simulink model "gm_spectrum_analyser"  (R2020a)
settings: Solver=VariableStepAuto  StartTime=0.0  StopTime=100000/256e6  RelTol=1e-3
InitFcn:
  | fs = 256e6;
undefined symbols (not defined in the file or in its folder): designMultirateFIR
libraries: hdlsllib x81, simulink x50, dspmlti4 x6, dsphdlxfrm x5, hdlmdlgenlib x4, dspswit3 x4, dspsigops x2, dspsigattribs x2
(part 4 of 5)

== system gm_spectrum_analyser/Spectrum Analyser/Spectrum Analyser/Spectrum Analyser Core/Preprocessing Window/Direct Memory Access/DDR Read Controller ==
  length_in : Inport  OutDataTypeStr=uint32  PortDimensions=1  SampleTime=3.90625e-09
  address : Inport  Port=2  OutDataTypeStr=uint32  PortDimensions=1  SampleTime=3.90625e-09
  start : Inport  Port=3  OutDataTypeStr=boolean  PortDimensions=1  SampleTime=3.90625e-09
  rd_aready : Inport  Port=4  OutDataTypeStr=boolean  PortDimensions=1  SampleTime=3.90625e-09
  rd_dvalid : Inport  Port=5  OutDataTypeStr=boolean  PortDimensions=1  SampleTime=3.90625e-09
  slib_spectrum_analyser_c5_DDR_Read_Controller : MATLAB Function  TreatAsAtomicUnit=on
  valid_out : Outport  VectorParamsAs1DForOutWhenUnconnected=off
  count_out : Outport  Port=2  VectorParamsAs1DForOutWhenUnconnected=off
  ready_out : Outport  Port=3  VectorParamsAs1DForOutWhenUnconnected=off
  rd_addr : Outport  Port=4  VectorParamsAs1DForOutWhenUnconnected=off
  rd_len : Outport  Port=5  VectorParamsAs1DForOutWhenUnconnected=off
  rd_avalid : Outport  Port=6  VectorParamsAs1DForOutWhenUnconnected=off
  wires:
  slib_spectrum_analyser_c5_DDR_Read_Controller/1(valid_out) -> valid_out/1
  slib_spectrum_analyser_c5_DDR_Read_Controller/2(count_out) -> count_out/1
  slib_spectrum_analyser_c5_DDR_Read_Controller/3(ready_out) -> ready_out/1
  slib_spectrum_analyser_c5_DDR_Read_Controller/4(rd_addr) -> rd_addr/1
  slib_spectrum_analyser_c5_DDR_Read_Controller/5(rd_len) -> rd_len/1
  slib_spectrum_analyser_c5_DDR_Read_Controller/6(rd_avalid) -> rd_avalid/1
  length_in/1 -> slib_spectrum_analyser_c5_DDR_Read_Controller/1(length_in)
  address/1 -> slib_spectrum_analyser_c5_DDR_Read_Controller/2(address)
  start/1 -> slib_spectrum_analyser_c5_DDR_Read_Controller/3(start)
  rd_aready/1 -> slib_spectrum_analyser_c5_DDR_Read_Controller/4(rd_aready)
  rd_dvalid/1 -> slib_spectrum_analyser_c5_DDR_Read_Controller/5(rd_dvalid)

== system gm_spectrum_analyser/Spectrum Analyser/Spectrum Analyser/Spectrum Analyser Core/Preprocessing Window/Direct Memory Access/EdgeDetection ==
  In1 : Inport  OutDataTypeStr=fixdt(0, 1, 0)  PortDimensions=1  SampleTime=3.90625e-09
  Delay : Delay  DelayLength=double(1)  InitialCondition=0  SampleTime=3.90625e-09
  Logical Operator : Logic  AllPortsSameDT=off  OutDataTypeStr=boolean  SampleTime=3.90625e-09
  Logical Operator1 : Logic  Operator=NOT  Inputs=1  AllPortsSameDT=off  OutDataTypeStr=boolean  SampleTime=3.90625e-09
  Out1 : Outport  VectorParamsAs1DForOutWhenUnconnected=off
  wires:
  Delay/1 -> Logical Operator1/1
  Logical Operator/1 -> Out1/1
  Logical Operator1/1 -> Logical Operator/1
  In1/1 -> Logical Operator/2, Delay/1

== system gm_spectrum_analyser/Spectrum Analyser/Spectrum Analyser/Spectrum Analyser Core/SSR Subset Converter/SSR Deserializer Imag/SSR to Vector ==
  SSR : Inport  OutDataTypeStr=fixdt(0, 128, 0)  PortDimensions=1  SampleTime=3.90625e-09
  Bit Slice0 : hdlsllib/Logic and Bit Operations/Bit Slice  lidx=double(15)  ridx=double(0)
      settings: SourceProductBaseCode=SL
  Bit Slice1 : hdlsllib/Logic and Bit Operations/Bit Slice  lidx=double(31)  ridx=double(16)
      settings: SourceProductBaseCode=SL
  Bit Slice2 : hdlsllib/Logic and Bit Operations/Bit Slice  lidx=double(47)  ridx=double(32)
      settings: SourceProductBaseCode=SL
  Bit Slice3 : hdlsllib/Logic and Bit Operations/Bit Slice  lidx=double(63)  ridx=double(48)
      settings: SourceProductBaseCode=SL
  Bit Slice4 : hdlsllib/Logic and Bit Operations/Bit Slice  lidx=double(79)  ridx=double(64)
      settings: SourceProductBaseCode=SL
  Bit Slice5 : hdlsllib/Logic and Bit Operations/Bit Slice  lidx=double(95)  ridx=double(80)
      settings: SourceProductBaseCode=SL
  Bit Slice6 : hdlsllib/Logic and Bit Operations/Bit Slice  lidx=double(111)  ridx=double(96)
      settings: SourceProductBaseCode=SL
  Bit Slice7 : hdlsllib/Logic and Bit Operations/Bit Slice  lidx=double(127)  ridx=double(112)
      settings: SourceProductBaseCode=SL
  concatenate : Concatenate  NumInputs=8
  Vector : Outport
  wires:
  Bit Slice0/1 -> concatenate/1
  Bit Slice1/1 -> concatenate/2
  Bit Slice2/1 -> concatenate/3
  Bit Slice3/1 -> concatenate/4
  Bit Slice4/1 -> concatenate/5
  Bit Slice5/1 -> concatenate/6
  Bit Slice6/1 -> concatenate/7
  Bit Slice7/1 -> concatenate/8
  concatenate/1 -> Vector/1
  SSR/1 -> Bit Slice7/1, Bit Slice6/1, Bit Slice5/1, Bit Slice4/1, Bit Slice3/1, Bit Slice2/1, Bit Slice1/1, Bit Slice0/1

== system gm_spectrum_analyser/Spectrum Analyser/Spectrum Analyser/Spectrum Analyser Core/SSR Subset Converter/SSR Deserializer Imag/Subsystem ==
  Set : Inport  OutDataTypeStr=boolean  PortDimensions=1  SampleTime=3.90625e-09
  Reset : Inport  Port=2  OutDataTypeStr=boolean  PortDimensions=1  SampleTime=3.90625e-09
  Constant : Constant  OutDataTypeStr=boolean  SampleTime=3.90625e-09
  Initial_Val : Constant  Value=double(0)  OutDataTypeStr=boolean  SampleTime=3.90625e-09
  Multiport Switch : MultiPortSwitch  DataPortOrder=Zero-based contiguous  Inputs=2  DiagnosticForDefault=None  zeroidx=on  SampleTime=3.90625e-09
  Unit Delay Resettable Synchronous_lowered : Delay  DelayLength=double(1)  InitialCondition=0  SampleTime=3.90625e-09
  reset_in : Switch  Criteria=u2 ~= 0  Threshold=double(0)  OutDataTypeStr=boolean  SampleTime=3.90625e-09
  Latch : Outport
  wires:
  Constant/1 -> Multiport Switch/3
  Multiport Switch/1 -> Latch/1, reset_in/3
  Initial_Val/1 -> reset_in/1
  Set/1 -> Multiport Switch/1
  Reset/1 -> reset_in/2
  reset_in/1 -> Unit Delay Resettable Synchronous_lowered/1
  Unit Delay Resettable Synchronous_lowered/1 -> Multiport Switch/2

== system gm_spectrum_analyser/Spectrum Analyser/Spectrum Analyser/Spectrum Analyser Core/SSR Subset Converter/SSR Deserializer Imag/Subsystem1 ==
  Set : Inport  OutDataTypeStr=boolean  PortDimensions=1  SampleTime=3.90625e-09
  Reset : Inport  Port=2  OutDataTypeStr=boolean  PortDimensions=1  SampleTime=3.90625e-09
  Constant : Constant  OutDataTypeStr=boolean  SampleTime=3.90625e-09
  Initial_Val : Constant  Value=double(0)  OutDataTypeStr=boolean  SampleTime=3.90625e-09
  Multiport Switch : MultiPortSwitch  DataPortOrder=Zero-based contiguous  Inputs=2  DiagnosticForDefault=None  zeroidx=on  SampleTime=3.90625e-09
  Unit Delay Resettable Synchronous_lowered : Delay  DelayLength=double(1)  InitialCondition=0  SampleTime=3.90625e-09
  reset_in : Switch  Criteria=u2 ~= 0  Threshold=double(0)  OutDataTypeStr=boolean  SampleTime=3.90625e-09
  Latch : Outport
  wires:
  Constant/1 -> Multiport Switch/3
  Multiport Switch/1 -> Latch/1, reset_in/3
  Initial_Val/1 -> reset_in/1
  Set/1 -> Multiport Switch/1
  Reset/1 -> reset_in/2
  reset_in/1 -> Unit Delay Resettable Synchronous_lowered/1
  Unit Delay Resettable Synchronous_lowered/1 -> Multiport Switch/2

== system gm_spectrum_analyser/Spectrum Analyser/Spectrum Analyser/Spectrum Analyser Core/SSR Subset Converter/SSR Deserializer Real/SSR to Vector ==
  SSR : Inport  OutDataTypeStr=fixdt(0, 128, 0)  PortDimensions=1  SampleTime=3.90625e-09
  Bit Slice0 : hdlsllib/Logic and Bit Operations/Bit Slice  lidx=double(15)  ridx=double(0)
      settings: SourceProductBaseCode=SL
  Bit Slice1 : hdlsllib/Logic and Bit Operations/Bit Slice  lidx=double(31)  ridx=double(16)
      settings: SourceProductBaseCode=SL
  Bit Slice2 : hdlsllib/Logic and Bit Operations/Bit Slice  lidx=double(47)  ridx=double(32)
      settings: SourceProductBaseCode=SL
  Bit Slice3 : hdlsllib/Logic and Bit Operations/Bit Slice  lidx=double(63)  ridx=double(48)
      settings: SourceProductBaseCode=SL
  Bit Slice4 : hdlsllib/Logic and Bit Operations/Bit Slice  lidx=double(79)  ridx=double(64)
      settings: SourceProductBaseCode=SL
  Bit Slice5 : hdlsllib/Logic and Bit Operations/Bit Slice  lidx=double(95)  ridx=double(80)
      settings: SourceProductBaseCode=SL
  Bit Slice6 : hdlsllib/Logic and Bit Operations/Bit Slice  lidx=double(111)  ridx=double(96)
      settings: SourceProductBaseCode=SL
  Bit Slice7 : hdlsllib/Logic and Bit Operations/Bit Slice  lidx=double(127)  ridx=double(112)
      settings: SourceProductBaseCode=SL
  concatenate : Concatenate  NumInputs=8
  Vector : Outport
  wires:
  Bit Slice0/1 -> concatenate/1
  Bit Slice1/1 -> concatenate/2
  Bit Slice2/1 -> concatenate/3
  Bit Slice3/1 -> concatenate/4
  Bit Slice4/1 -> concatenate/5
  Bit Slice5/1 -> concatenate/6
  Bit Slice6/1 -> concatenate/7
  Bit Slice7/1 -> concatenate/8
  concatenate/1 -> Vector/1
  SSR/1 -> Bit Slice7/1, Bit Slice6/1, Bit Slice5/1, Bit Slice4/1, Bit Slice3/1, Bit Slice2/1, Bit Slice1/1, Bit Slice0/1

== system gm_spectrum_analyser/Spectrum Analyser/Spectrum Analyser/Spectrum Analyser Core/SSR Subset Converter/SSR Deserializer Real/Subsystem ==
  Set : Inport  OutDataTypeStr=boolean  PortDimensions=1  SampleTime=3.90625e-09
  Reset : Inport  Port=2  OutDataTypeStr=boolean  PortDimensions=1  SampleTime=3.90625e-09
  Constant : Constant  OutDataTypeStr=boolean  SampleTime=3.90625e-09
  Initial_Val : Constant  Value=double(0)  OutDataTypeStr=boolean  SampleTime=3.90625e-09
  Multiport Switch : MultiPortSwitch  DataPortOrder=Zero-based contiguous  Inputs=2  DiagnosticForDefault=None  zeroidx=on  SampleTime=3.90625e-09
  Unit Delay Resettable Synchronous_lowered : Delay  DelayLength=double(1)  InitialCondition=0  SampleTime=3.90625e-09
  reset_in : Switch  Criteria=u2 ~= 0  Threshold=double(0)  OutDataTypeStr=boolean  SampleTime=3.90625e-09
  Latch : Outport
  wires:
  Constant/1 -> Multiport Switch/3
  Multiport Switch/1 -> Latch/1, reset_in/3
  Initial_Val/1 -> reset_in/1
  Set/1 -> Multiport Switch/1
  Reset/1 -> reset_in/2
  reset_in/1 -> Unit Delay Resettable Synchronous_lowered/1
  Unit Delay Resettable Synchronous_lowered/1 -> Multiport Switch/2

== system gm_spectrum_analyser/Spectrum Analyser/Spectrum Analyser/Spectrum Analyser Core/SSR Subset Converter/SSR Deserializer Real/Subsystem1 ==
  Set : Inport  OutDataTypeStr=boolean  PortDimensions=1  SampleTime=3.90625e-09
  Reset : Inport  Port=2  OutDataTypeStr=boolean  PortDimensions=1  SampleTime=3.90625e-09
  Constant : Constant  OutDataTypeStr=boolean  SampleTime=3.90625e-09
  Initial_Val : Constant  Value=double(0)  OutDataTypeStr=boolean  SampleTime=3.90625e-09
  Multiport Switch : MultiPortSwitch  DataPortOrder=Zero-based contiguous  Inputs=2  DiagnosticForDefault=None  zeroidx=on  SampleTime=3.90625e-09
  Unit Delay Resettable Synchronous_lowered : Delay  DelayLength=double(1)  InitialCondition=0  SampleTime=3.90625e-09
  reset_in : Switch  Criteria=u2 ~= 0  Threshold=double(0)  OutDataTypeStr=boolean  SampleTime=3.90625e-09
  Latch : Outport
  wires:
  Constant/1 -> Multiport Switch/3
  Multiport Switch/1 -> Latch/1, reset_in/3
  Initial_Val/1 -> reset_in/1
  Set/1 -> Multiport Switch/1
  Reset/1 -> reset_in/2
  reset_in/1 -> Unit Delay Resettable Synchronous_lowered/1
  Unit Delay Resettable Synchronous_lowered/1 -> Multiport Switch/2

== system gm_spectrum_analyser/Spectrum Analyser/Spectrum Analyser/Spectrum Analyser Core/SSR Subset Converter/SSR Packet Generator Imag/Frame Dropper ==
  Valid In : Inport  OutDataTypeStr=boolean  PortDimensions=1  SampleTime=3.90625e-09
  Data In : Inport  Port=2  OutDataTypeStr=fixdt(0, 128, 0)  PortDimensions=1  SampleTime=3.90625e-09
  SoF In : Inport  Port=3  OutDataTypeStr=boolean  PortDimensions=1  SampleTime=3.90625e-09
  EoF In : Inport  Port=4  OutDataTypeStr=boolean  PortDimensions=1  SampleTime=3.90625e-09
  Frame Drop : Inport  Port=5  OutDataTypeStr=fixdt(0, 4, 0)  PortDimensions=1  SampleTime=3.90625e-09
  AND : Logic  AllPortsSameDT=off  OutDataTypeStr=boolean  SampleTime=3.90625e-09
  AND1 : Logic  AllPortsSameDT=off  OutDataTypeStr=boolean  SampleTime=3.90625e-09
  AND2 : Logic  AllPortsSameDT=off  OutDataTypeStr=boolean  SampleTime=3.90625e-09
  Compare To Zero : simulink/Logic and Bit Operations/Compare To Constant  relop===  const=double(0)  OutDataTypeStr=boolean
  Constant : Constant  Value=0  OutDataTypeStr=fixdt(0, 4, 0)  SampleTime=3.90625e-09
  Constant1 : Constant  OutDataTypeStr=fixdt(0, 4, 0)  SampleTime=3.90625e-09
  HDL Counter : hdlsllib/Sources/HDL Counter  CountType=Count limited  CountInit=double(0)  CountStep=double(1)  CountMax=double(7)  CountFromType=Initial value  CountFrom=double(0)  CountResetPort=on  CountLoadPort=off  CountEnbPort=on  CountDirPort=off  CountDataType=Unsigned  CountWordLen=4  CountFracLen=0  CountSampTime=3.90625e-09
  Multiport Switch : MultiPortSwitch  DataPortOrder=Zero-based contiguous  Inputs=2  DiagnosticForDefault=None  zeroidx=on  OutDataTypeStr=fixdt(0, 4, 0)  SampleTime=3.90625e-09
  Relational Operator : RelationalOperator  Operator=<=  OutDataTypeStr=boolean  SampleTime=3.90625e-09  RndMeth=Nearest
  shift arithmetic : ArithShift  BitShiftNumberSource=Input port  BitShiftDirection=Left
      settings: InputPortMap=u0,p1
  Valid Out : Outport
  Data Out : Outport  Port=2
  SoF Out : Outport  Port=3
  EoF Out : Outport  Port=4
  wires:
  AND/1 -> Valid Out/1
  AND1/1 -> EoF Out/1
  AND2/1 -> SoF Out/1
  Compare To Zero/1 -> AND2/1, AND1/1, AND/2
  Constant/1 -> Multiport Switch/3
  Constant1/1 -> shift arithmetic/1
  HDL Counter/1 -> Multiport Switch/2, Relational Operator/2
  Multiport Switch/1 -> Compare To Zero/1
  Relational Operator/1 -> Multiport Switch/1, HDL Counter/1
  shift arithmetic/1 -> Relational Operator/1
  Valid In/1 -> AND/1
  Data In/1 -> Data Out/1
  SoF In/1 -> AND2/2
  EoF In/1 -> AND1/2, HDL Counter/2
  Frame Drop/1 -> shift arithmetic/2

== system gm_spectrum_analyser/Spectrum Analyser/Spectrum Analyser/Spectrum Analyser Core/SSR Subset Converter/SSR Packet Generator Imag/TLAST Generator ==
  Valid In : Inport  OutDataTypeStr=boolean  PortDimensions=1  SampleTime=3.90625e-09
  Data In : Inport  Port=2  OutDataTypeStr=fixdt(0, 128, 0)  PortDimensions=1  SampleTime=3.90625e-09
  Packet Size : Inport  Port=3  OutDataTypeStr=uint32  PortDimensions=1  SampleTime=3.90625e-09
  AND : Logic  Inputs=3  AllPortsSameDT=off  OutDataTypeStr=boolean  SampleTime=3.90625e-09
  AND1 : Logic  Inputs=3  AllPortsSameDT=off  OutDataTypeStr=boolean  SampleTime=3.90625e-09
  AND2 : Logic  AllPortsSameDT=off  OutDataTypeStr=boolean  SampleTime=3.90625e-09
  AND3 : Logic  AllPortsSameDT=off  OutDataTypeStr=boolean  SampleTime=3.90625e-09
  Compare To Constant : simulink/Logic and Bit Operations/Compare To Constant  relop===  const="fi(0,0,32,0,\"hex\",\"00000001\")"  OutDataTypeStr=boolean
  Compare To Zero : simulink/Logic and Bit Operations/Compare To Constant  relop=~=  const=double(0)  OutDataTypeStr=boolean
  Delay_Switch : Switch  Criteria=u2 ~= 0  Threshold=double(0)  OutDataTypeStr=uint32  SampleTime=3.90625e-09
  HDL Counter : hdlsllib/Sources/HDL Counter  CountType=Free running  CountInit=double(1)  CountStep=double(1)  CountMax=25  CountFromType=Initial value  CountFrom=double(1)  CountResetPort=on  CountLoadPort=off  CountEnbPort=on  CountDirPort=off  CountDataType=Unsigned  CountWordLen=32  CountFracLen=0  CountSampTime=3.90625e-09
  Relational Operator : RelationalOperator  Operator=<=  OutDataTypeStr=boolean  SampleTime=3.90625e-09  RndMeth=Nearest
  Unit Delay Enabled Synchronous_lowered : Delay  DelayLength=double(1)  InitialCondition=0  SampleTime=3.90625e-09
  Valid Out : Outport
  Data Out : Outport  Port=2
  SoF Out : Outport  Port=3
  EoF Out : Outport  Port=4
  wires:
  AND/1 -> SoF Out/1
  AND1/1 -> EoF Out/1, HDL Counter/1
  AND2/1 -> Valid Out/1
  Compare To Constant/1 -> AND/1
  Compare To Zero/1 -> AND2/1, AND/3, AND1/3
  HDL Counter/1 -> Compare To Constant/1, Relational Operator/2
  Valid In/1 -> AND2/2, AND/2, AND3/1, AND1/2, HDL Counter/2
  Data In/1 -> Data Out/1
  Packet Size/1 -> Delay_Switch/1
  Relational Operator/1 -> AND3/2, AND1/1
  AND3/1 -> Delay_Switch/2
  Delay_Switch/1 -> Unit Delay Enabled Synchronous_lowered/1
  Unit Delay Enabled Synchronous_lowered/1 -> Relational Operator/1, Compare To Zero/1, Delay_Switch/3

== system gm_spectrum_analyser/Spectrum Analyser/Spectrum Analyser/Spectrum Analyser Core/SSR Subset Converter/SSR Packet Generator Real/Frame Dropper ==
  Valid In : Inport  OutDataTypeStr=boolean  PortDimensions=1  SampleTime=3.90625e-09
  Data In : Inport  Port=2  OutDataTypeStr=fixdt(0, 128, 0)  PortDimensions=1  SampleTime=3.90625e-09
  SoF In : Inport  Port=3  OutDataTypeStr=boolean  PortDimensions=1  SampleTime=3.90625e-09
  EoF In : Inport  Port=4  OutDataTypeStr=boolean  PortDimensions=1  SampleTime=3.90625e-09
  Frame Drop : Inport  Port=5  OutDataTypeStr=fixdt(0, 4, 0)  PortDimensions=1  SampleTime=3.90625e-09
  AND : Logic  AllPortsSameDT=off  OutDataTypeStr=boolean  SampleTime=3.90625e-09
  AND1 : Logic  AllPortsSameDT=off  OutDataTypeStr=boolean  SampleTime=3.90625e-09
  AND2 : Logic  AllPortsSameDT=off  OutDataTypeStr=boolean  SampleTime=3.90625e-09
  Compare To Zero : simulink/Logic and Bit Operations/Compare To Constant  relop===  const=double(0)  OutDataTypeStr=boolean
  Constant : Constant  Value=0  OutDataTypeStr=fixdt(0, 4, 0)  SampleTime=3.90625e-09
  Constant1 : Constant  OutDataTypeStr=fixdt(0, 4, 0)  SampleTime=3.90625e-09
  HDL Counter : hdlsllib/Sources/HDL Counter  CountType=Count limited  CountInit=double(0)  CountStep=double(1)  CountMax=double(7)  CountFromType=Initial value  CountFrom=double(0)  CountResetPort=on  CountLoadPort=off  CountEnbPort=on  CountDirPort=off  CountDataType=Unsigned  CountWordLen=4  CountFracLen=0  CountSampTime=3.90625e-09
  Multiport Switch : MultiPortSwitch  DataPortOrder=Zero-based contiguous  Inputs=2  DiagnosticForDefault=None  zeroidx=on  OutDataTypeStr=fixdt(0, 4, 0)  SampleTime=3.90625e-09
  Relational Operator : RelationalOperator  Operator=<=  OutDataTypeStr=boolean  SampleTime=3.90625e-09  RndMeth=Nearest
  shift arithmetic : ArithShift  BitShiftNumberSource=Input port  BitShiftDirection=Left
      settings: InputPortMap=u0,p1
  Valid Out : Outport
  Data Out : Outport  Port=2
  SoF Out : Outport  Port=3
  EoF Out : Outport  Port=4
  wires:
  AND/1 -> Valid Out/1
  AND1/1 -> EoF Out/1
  AND2/1 -> SoF Out/1
  Compare To Zero/1 -> AND2/1, AND1/1, AND/2
  Constant/1 -> Multiport Switch/3
  Constant1/1 -> shift arithmetic/1
  HDL Counter/1 -> Multiport Switch/2, Relational Operator/2
  Multiport Switch/1 -> Compare To Zero/1
  Relational Operator/1 -> Multiport Switch/1, HDL Counter/1
  shift arithmetic/1 -> Relational Operator/1
  Valid In/1 -> AND/1
  Data In/1 -> Data Out/1
  SoF In/1 -> AND2/2
  EoF In/1 -> AND1/2, HDL Counter/2
  Frame Drop/1 -> shift arithmetic/2

== system gm_spectrum_analyser/Spectrum Analyser/Spectrum Analyser/Spectrum Analyser Core/SSR Subset Converter/SSR Packet Generator Real/TLAST Generator ==
  Valid In : Inport  OutDataTypeStr=boolean  PortDimensions=1  SampleTime=3.90625e-09
  Data In : Inport  Port=2  OutDataTypeStr=fixdt(0, 128, 0)  PortDimensions=1  SampleTime=3.90625e-09
  Packet Size : Inport  Port=3  OutDataTypeStr=uint32  PortDimensions=1  SampleTime=3.90625e-09
  AND : Logic  Inputs=3  AllPortsSameDT=off  OutDataTypeStr=boolean  SampleTime=3.90625e-09
  AND1 : Logic  Inputs=3  AllPortsSameDT=off  OutDataTypeStr=boolean  SampleTime=3.90625e-09
  AND2 : Logic  AllPortsSameDT=off  OutDataTypeStr=boolean  SampleTime=3.90625e-09
  AND3 : Logic  AllPortsSameDT=off  OutDataTypeStr=boolean  SampleTime=3.90625e-09
  Compare To Constant : simulink/Logic and Bit Operations/Compare To Constant  relop===  const="fi(0,0,32,0,\"hex\",\"00000001\")"  OutDataTypeStr=boolean
  Compare To Zero : simulink/Logic and Bit Operations/Compare To Constant  relop=~=  const=double(0)  OutDataTypeStr=boolean
  Delay_Switch : Switch  Criteria=u2 ~= 0  Threshold=double(0)  OutDataTypeStr=uint32  SampleTime=3.90625e-09
  HDL Counter : hdlsllib/Sources/HDL Counter  CountType=Free running  CountInit=double(1)  CountStep=double(1)  CountMax=25  CountFromType=Initial value  CountFrom=double(1)  CountResetPort=on  CountLoadPort=off  CountEnbPort=on  CountDirPort=off  CountDataType=Unsigned  CountWordLen=32  CountFracLen=0  CountSampTime=3.90625e-09
  Relational Operator : RelationalOperator  Operator=<=  OutDataTypeStr=boolean  SampleTime=3.90625e-09  RndMeth=Nearest
  Unit Delay Enabled Synchronous_lowered : Delay  DelayLength=double(1)  InitialCondition=0  SampleTime=3.90625e-09
  Valid Out : Outport
  Data Out : Outport  Port=2
  SoF Out : Outport  Port=3
  EoF Out : Outport  Port=4
  wires:
  AND/1 -> SoF Out/1
  AND1/1 -> EoF Out/1, HDL Counter/1
  AND2/1 -> Valid Out/1
  Compare To Constant/1 -> AND/1
  Compare To Zero/1 -> AND2/1, AND/3, AND1/3
  HDL Counter/1 -> Compare To Constant/1, Relational Operator/2
  Valid In/1 -> AND2/2, AND/2, AND3/1, AND1/2, HDL Counter/2
  Data In/1 -> Data Out/1
  Packet Size/1 -> Delay_Switch/1
  Relational Operator/1 -> AND3/2, AND1/1
  AND3/1 -> Delay_Switch/2
  Delay_Switch/1 -> Unit Delay Enabled Synchronous_lowered/1
  Unit Delay Enabled Synchronous_lowered/1 -> Relational Operator/1, Compare To Zero/1, Delay_Switch/3

== system gm_spectrum_analyser/Spectrum Analyser/Spectrum Analyser/Spectrum Analyser Core/SSR Subset Converter/SSR Serializer Imag/SSR to Vector ==
  SSR : Inport  OutDataTypeStr=fixdt(0, 128, 0)  PortDimensions=1  SampleTime=3.90625e-09
  Bit Slice0 : hdlsllib/Logic and Bit Operations/Bit Slice  lidx=double(15)  ridx=double(0)
      settings: SourceProductBaseCode=SL
  Bit Slice1 : hdlsllib/Logic and Bit Operations/Bit Slice  lidx=double(31)  ridx=double(16)
      settings: SourceProductBaseCode=SL
  Bit Slice2 : hdlsllib/Logic and Bit Operations/Bit Slice  lidx=double(47)  ridx=double(32)
      settings: SourceProductBaseCode=SL
  Bit Slice3 : hdlsllib/Logic and Bit Operations/Bit Slice  lidx=double(63)  ridx=double(48)
      settings: SourceProductBaseCode=SL
  Bit Slice4 : hdlsllib/Logic and Bit Operations/Bit Slice  lidx=double(79)  ridx=double(64)
      settings: SourceProductBaseCode=SL
  Bit Slice5 : hdlsllib/Logic and Bit Operations/Bit Slice  lidx=double(95)  ridx=double(80)
      settings: SourceProductBaseCode=SL
  Bit Slice6 : hdlsllib/Logic and Bit Operations/Bit Slice  lidx=double(111)  ridx=double(96)
      settings: SourceProductBaseCode=SL
  Bit Slice7 : hdlsllib/Logic and Bit Operations/Bit Slice  lidx=double(127)  ridx=double(112)
      settings: SourceProductBaseCode=SL
  concatenate : Concatenate  NumInputs=8
  Vector : Outport
  wires:
  Bit Slice0/1 -> concatenate/1
  Bit Slice1/1 -> concatenate/2
  Bit Slice2/1 -> concatenate/3
  Bit Slice3/1 -> concatenate/4
  Bit Slice4/1 -> concatenate/5
  Bit Slice5/1 -> concatenate/6
  Bit Slice6/1 -> concatenate/7
  Bit Slice7/1 -> concatenate/8
  concatenate/1 -> Vector/1
  SSR/1 -> Bit Slice7/1, Bit Slice6/1, Bit Slice5/1, Bit Slice4/1, Bit Slice3/1, Bit Slice2/1, Bit Slice1/1, Bit Slice0/1

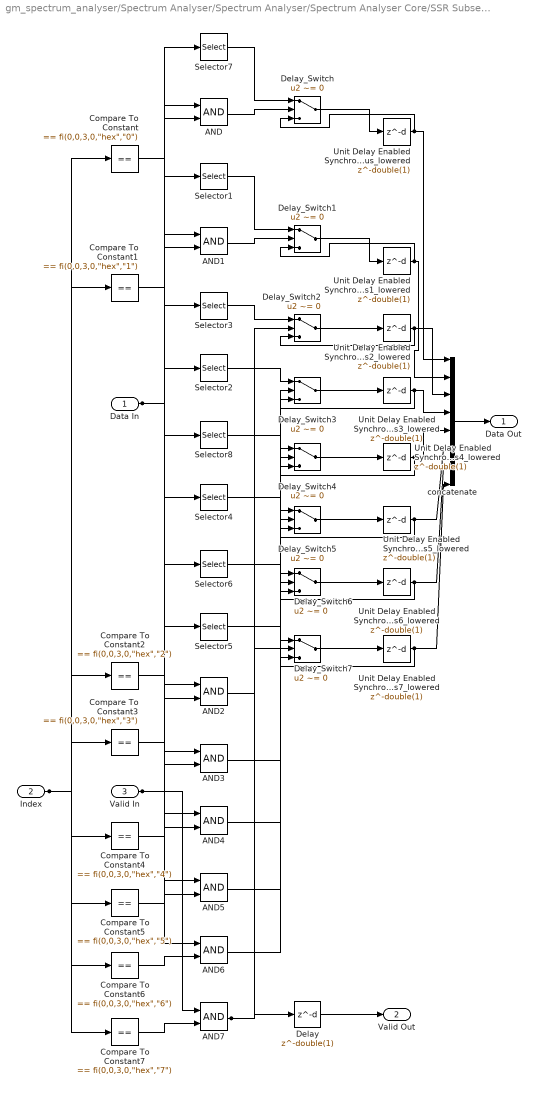
== system gm_spectrum_analyser/Spectrum Analyser/Spectrum Analyser/Spectrum Analyser Core/SSR Subset Converter/SSR Serializer Imag/SSR1 to SSR8 ==
  Data In : Inport  OutDataTypeStr=uint16  PortDimensions=[8]  SampleTime=3.90625e-09
  Index : Inport  Port=2  OutDataTypeStr=fixdt(0, 3, 0)  PortDimensions=1  SampleTime=3.90625e-09
  Valid In : Inport  Port=3  OutDataTypeStr=boolean  PortDimensions=1  SampleTime=3.90625e-09
  AND{,1..7} (8 alike) : Logic  AllPortsSameDT=off  OutDataTypeStr=boolean  SampleTime=3.90625e-09
  Compare To Constant : simulink/Logic and Bit Operations/Compare To Constant  relop===  const="fi(0,0,3,0,\"hex\",\"0\")"  OutDataTypeStr=boolean
  Compare To Constant1 : simulink/Logic and Bit Operations/Compare To Constant  relop===  const="fi(0,0,3,0,\"hex\",\"1\")"  OutDataTypeStr=boolean
  Compare To Constant2 : simulink/Logic and Bit Operations/Compare To Constant  relop===  const="fi(0,0,3,0,\"hex\",\"2\")"  OutDataTypeStr=boolean
  Compare To Constant3 : simulink/Logic and Bit Operations/Compare To Constant  relop===  const="fi(0,0,3,0,\"hex\",\"3\")"  OutDataTypeStr=boolean
  Compare To Constant4 : simulink/Logic and Bit Operations/Compare To Constant  relop===  const="fi(0,0,3,0,\"hex\",\"4\")"  OutDataTypeStr=boolean
  Compare To Constant5 : simulink/Logic and Bit Operations/Compare To Constant  relop===  const="fi(0,0,3,0,\"hex\",\"5\")"  OutDataTypeStr=boolean
  Compare To Constant6 : simulink/Logic and Bit Operations/Compare To Constant  relop===  const="fi(0,0,3,0,\"hex\",\"6\")"  OutDataTypeStr=boolean
  Compare To Constant7 : simulink/Logic and Bit Operations/Compare To Constant  relop===  const="fi(0,0,3,0,\"hex\",\"7\")"  OutDataTypeStr=boolean
  Delay : Delay  DelayLength=double(1)  InitialCondition=0  SampleTime=3.90625e-09
  Delay_Switch{,1..7} (8 alike) : Switch  Criteria=u2 ~= 0  Threshold=double(0)  OutDataTypeStr=uint16  SampleTime=3.90625e-09
  Selector{1..8} (8 alike) : Selector  IndexMode=Zero-based  SampleTime=3.90625e-09  IndexOptions=Index vector (dialog)  Indices=double(0)  OutputSizes=double(1)
  Unit Delay Enabled Synchronous1_lowered : Delay  DelayLength=double(1)  InitialCondition=0  SampleTime=3.90625e-09
  Unit Delay Enabled Synchronous2_lowered : Delay  DelayLength=double(1)  InitialCondition=0  SampleTime=3.90625e-09
  Unit Delay Enabled Synchronous3_lowered : Delay  DelayLength=double(1)  InitialCondition=0  SampleTime=3.90625e-09
  Unit Delay Enabled Synchronous4_lowered : Delay  DelayLength=double(1)  InitialCondition=0  SampleTime=3.90625e-09
  Unit Delay Enabled Synchronous5_lowered : Delay  DelayLength=double(1)  InitialCondition=0  SampleTime=3.90625e-09
  Unit Delay Enabled Synchronous6_lowered : Delay  DelayLength=double(1)  InitialCondition=0  SampleTime=3.90625e-09
  Unit Delay Enabled Synchronous7_lowered : Delay  DelayLength=double(1)  InitialCondition=0  SampleTime=3.90625e-09
  Unit Delay Enabled Synchronous_lowered : Delay  DelayLength=double(1)  InitialCondition=0  SampleTime=3.90625e-09
  concatenate : Concatenate  NumInputs=8
  Data Out : Outport
  Valid Out : Outport  Port=2
  wires:
  AND/1 -> Delay_Switch/2
  AND1/1 -> Delay_Switch1/2
  AND2/1 -> Delay_Switch2/2
  AND3/1 -> Delay_Switch3/2
  AND4/1 -> Delay_Switch4/2
  AND5/1 -> Delay_Switch5/2
  AND6/1 -> Delay_Switch6/2
  AND7/1 -> Delay/1, Delay_Switch7/2
  Compare To Constant/1 -> AND/2
  Compare To Constant1/1 -> AND1/2
  Compare To Constant2/1 -> AND2/2
  Compare To Constant3/1 -> AND3/2
  Compare To Constant4/1 -> AND4/2
  Compare To Constant5/1 -> AND5/2
  Compare To Constant6/1 -> AND6/2
  Compare To Constant7/1 -> AND7/2
  Delay/1 -> Valid Out/1
  Selector1/1 -> Delay_Switch1/1
  Selector2/1 -> Delay_Switch3/1
  Selector3/1 -> Delay_Switch2/1
  Selector4/1 -> Delay_Switch5/1
  Selector5/1 -> Delay_Switch7/1
  Selector6/1 -> Delay_Switch6/1
  Selector7/1 -> Delay_Switch/1
  Selector8/1 -> Delay_Switch4/1
  Unit Delay Enabled Synchronous_lowered/1 -> concatenate/1, Delay_Switch/3
  Unit Delay Enabled Synchronous1_lowered/1 -> concatenate/2, Delay_Switch1/3
  Unit Delay Enabled Synchronous2_lowered/1 -> concatenate/3, Delay_Switch2/3
  Unit Delay Enabled Synchronous3_lowered/1 -> concatenate/4, Delay_Switch3/3
  Unit Delay Enabled Synchronous4_lowered/1 -> concatenate/5, Delay_Switch4/3
  Unit Delay Enabled Synchronous5_lowered/1 -> concatenate/6, Delay_Switch5/3
  Unit Delay Enabled Synchronous6_lowered/1 -> concatenate/7, Delay_Switch6/3
  Unit Delay Enabled Synchronous7_lowered/1 -> concatenate/8, Delay_Switch7/3
  concatenate/1 -> Data Out/1
  Data In/1 -> Selector8/1, Selector7/1, Selector6/1, Selector5/1, Selector4/1, Selector3/1, Selector2/1, Selector1/1
  Index/1 -> Compare To Constant7/1, Compare To Constant6/1, Compare To Constant5/1, Compare To Constant4/1, Compare To Constant3/1, Compare To Constant2/1, Compare To Constant1/1, Compare To Constant/1
  Valid In/1 -> AND7/1, AND6/1, AND5/1, AND4/1, AND3/1, AND2/1, AND1/1, AND/1
  Delay_Switch/1 -> Unit Delay Enabled Synchronous_lowered/1
  Delay_Switch1/1 -> Unit Delay Enabled Synchronous1_lowered/1
  Delay_Switch2/1 -> Unit Delay Enabled Synchronous2_lowered/1
  Delay_Switch3/1 -> Unit Delay Enabled Synchronous3_lowered/1
  Delay_Switch4/1 -> Unit Delay Enabled Synchronous4_lowered/1
  Delay_Switch5/1 -> Unit Delay Enabled Synchronous5_lowered/1
  Delay_Switch6/1 -> Unit Delay Enabled Synchronous6_lowered/1
  Delay_Switch7/1 -> Unit Delay Enabled Synchronous7_lowered/1

== system gm_spectrum_analyser/Spectrum Analyser/Spectrum Analyser/Spectrum Analyser Core/SSR Subset Converter/SSR Serializer Imag/SSR2 to SSR8 ==
  Data In : Inport  OutDataTypeStr=uint16  PortDimensions=[8]  SampleTime=3.90625e-09
  Index : Inport  Port=2  OutDataTypeStr=fixdt(0, 2, 0)  PortDimensions=1  SampleTime=3.90625e-09
  Valid In : Inport  Port=3  OutDataTypeStr=boolean  PortDimensions=1  SampleTime=3.90625e-09
  AND{,1..3} (4 alike) : Logic  AllPortsSameDT=off  OutDataTypeStr=boolean  SampleTime=3.90625e-09
  Compare To Constant10 : simulink/Logic and Bit Operations/Compare To Constant  relop===  const="fi(0,0,2,0,\"hex\",\"2\")"  OutDataTypeStr=boolean
  Compare To Constant11 : simulink/Logic and Bit Operations/Compare To Constant  relop===  const="fi(0,0,2,0,\"hex\",\"3\")"  OutDataTypeStr=boolean
  Compare To Constant8 : simulink/Logic and Bit Operations/Compare To Constant  relop===  const="fi(0,0,2,0,\"hex\",\"0\")"  OutDataTypeStr=boolean
  Compare To Constant9 : simulink/Logic and Bit Operations/Compare To Constant  relop===  const="fi(0,0,2,0,\"hex\",\"1\")"  OutDataTypeStr=boolean
  Delay : Delay  DelayLength=double(1)  InitialCondition=0  SampleTime=3.90625e-09
  Delay_Switch{,1..3} (4 alike) : Switch  Criteria=u2 ~= 0  Threshold=double(0)  OutDataTypeStr=uint16  SampleTime=3.90625e-09
  Selector{9..12} (4 alike) : Selector  IndexMode=Zero-based  SampleTime=3.90625e-09  IndexOptions=Index vector (dialog)  Indices=double([0 1])  OutputSizes=double(1)
  Unit Delay Enabled Synchronous1_lowered : Delay  DelayLength=double(1)  InitialCondition=0  SampleTime=3.90625e-09
  Unit Delay Enabled Synchronous2_lowered : Delay  DelayLength=double(1)  InitialCondition=0  SampleTime=3.90625e-09
  Unit Delay Enabled Synchronous3_lowered : Delay  DelayLength=double(1)  InitialCondition=0  SampleTime=3.90625e-09
  Unit Delay Enabled Synchronous_lowered : Delay  DelayLength=double(1)  InitialCondition=0  SampleTime=3.90625e-09
  concatenate : Concatenate  NumInputs=8
  t{,1..3} (4 alike) : Demux  Outputs=2
  Data Out : Outport
  Valid Out : Outport  Port=2
  wires:
  AND/1 -> Delay_Switch/2
  AND1/1 -> Delay_Switch1/2
  AND2/1 -> Delay_Switch2/2
  AND3/1 -> Delay/1, Delay_Switch3/2
  Compare To Constant10/1 -> AND2/2
  Compare To Constant11/1 -> AND3/2
  Compare To Constant8/1 -> AND/2
  Compare To Constant9/1 -> AND1/2
  Delay/1 -> Valid Out/1
  Selector10/1 -> Delay_Switch2/1
  Selector11/1 -> Delay_Switch3/1
  Selector12/1 -> Delay_Switch/1
  Selector9/1 -> Delay_Switch1/1
  Unit Delay Enabled Synchronous_lowered/1 -> t/1, Delay_Switch/3
  Unit Delay Enabled Synchronous1_lowered/1 -> t1/1, Delay_Switch1/3
  Unit Delay Enabled Synchronous2_lowered/1 -> t2/1, Delay_Switch2/3
  Unit Delay Enabled Synchronous3_lowered/1 -> t3/1, Delay_Switch3/3
  concatenate/1 -> Data Out/1
  t/1 -> concatenate/1
  t/2 -> concatenate/2
  t1/1 -> concatenate/3
  t1/2 -> concatenate/4
  t2/1 -> concatenate/5
  t2/2 -> concatenate/6
  t3/1 -> concatenate/7
  t3/2 -> concatenate/8
  Data In/1 -> Selector9/1, Selector12/1, Selector11/1, Selector10/1
  Index/1 -> Compare To Constant9/1, Compare To Constant8/1, Compare To Constant11/1, Compare To Constant10/1
  Valid In/1 -> AND3/1, AND2/1, AND1/1, AND/1
  Delay_Switch/1 -> Unit Delay Enabled Synchronous_lowered/1
  Delay_Switch1/1 -> Unit Delay Enabled Synchronous1_lowered/1
  Delay_Switch2/1 -> Unit Delay Enabled Synchronous2_lowered/1
  Delay_Switch3/1 -> Unit Delay Enabled Synchronous3_lowered/1

== system gm_spectrum_analyser/Spectrum Analyser/Spectrum Analyser/Spectrum Analyser Core/SSR Subset Converter/SSR Serializer Imag/SSR4 to SSR8 ==
  Data In : Inport  OutDataTypeStr=uint16  PortDimensions=[8]  SampleTime=3.90625e-09
  Index : Inport  Port=2  OutDataTypeStr=fixdt(0, 1, 0)  PortDimensions=1  SampleTime=3.90625e-09
  Valid In : Inport  Port=3  OutDataTypeStr=boolean  PortDimensions=1  SampleTime=3.90625e-09
  AND : Logic  AllPortsSameDT=off  OutDataTypeStr=boolean  SampleTime=3.90625e-09
  AND1 : Logic  AllPortsSameDT=off  OutDataTypeStr=boolean  SampleTime=3.90625e-09
  Compare To Constant12 : simulink/Logic and Bit Operations/Compare To Constant  relop===  const="fi(0,0,1,0,\"hex\",\"0\")"  OutDataTypeStr=boolean
  Compare To Constant13 : simulink/Logic and Bit Operations/Compare To Constant  relop===  const="fi(0,0,1,0,\"hex\",\"1\")"  OutDataTypeStr=boolean
  Delay : Delay  DelayLength=double(1)  InitialCondition=0  SampleTime=3.90625e-09
  Delay_Switch : Switch  Criteria=u2 ~= 0  Threshold=double(0)  OutDataTypeStr=uint16  SampleTime=3.90625e-09
  Delay_Switch1 : Switch  Criteria=u2 ~= 0  Threshold=double(0)  OutDataTypeStr=uint16  SampleTime=3.90625e-09
  Selector13 : Selector  IndexMode=Zero-based  SampleTime=3.90625e-09  IndexOptions=Index vector (dialog)  Indices=double([0 1 2 3])  OutputSizes=double(1)
  Selector14 : Selector  IndexMode=Zero-based  SampleTime=3.90625e-09  IndexOptions=Index vector (dialog)  Indices=double([0 1 2 3])  OutputSizes=double(1)
  Unit Delay Enabled Synchronous1_lowered : Delay  DelayLength=double(1)  InitialCondition=0  SampleTime=3.90625e-09
  Unit Delay Enabled Synchronous_lowered : Delay  DelayLength=double(1)  InitialCondition=0  SampleTime=3.90625e-09
  concatenate : Concatenate  NumInputs=8
  t : Demux
  t1 : Demux
  Data Out : Outport
  Valid Out : Outport  Port=2
  wires:
  AND/1 -> Delay_Switch/2
  AND1/1 -> Delay/1, Delay_Switch1/2
  Compare To Constant12/1 -> AND/2
  Compare To Constant13/1 -> AND1/2
  Delay/1 -> Valid Out/1
  Selector13/1 -> Delay_Switch/1
  Selector14/1 -> Delay_Switch1/1
  Unit Delay Enabled Synchronous_lowered/1 -> t/1, Delay_Switch/3
  Unit Delay Enabled Synchronous1_lowered/1 -> t1/1, Delay_Switch1/3
  concatenate/1 -> Data Out/1
  t/1 -> concatenate/1
  t/2 -> concatenate/2
  t/3 -> concatenate/3
  t/4 -> concatenate/4
  t1/1 -> concatenate/5
  t1/2 -> concatenate/6
  t1/3 -> concatenate/7
  t1/4 -> concatenate/8
  Data In/1 -> Selector14/1, Selector13/1
  Index/1 -> Compare To Constant13/1, Compare To Constant12/1
  Valid In/1 -> AND1/1, AND/1
  Delay_Switch/1 -> Unit Delay Enabled Synchronous_lowered/1
  Delay_Switch1/1 -> Unit Delay Enabled Synchronous1_lowered/1

== system gm_spectrum_analyser/Spectrum Analyser/Spectrum Analyser/Spectrum Analyser Core/SSR Subset Converter/SSR Serializer Imag/Vector to SSR ==
  Vector : Inport  OutDataTypeStr=uint16  PortDimensions=[8]  SampleTime=3.90625e-09
  Bit Concat : hdlsllib/Logic and Bit Operations/Bit Concat  numInputs=8
  Selector0 : Selector  SampleTime=3.90625e-09  IndexOptions=Index vector (dialog)  Indices=double(8)  OutputSizes=double(1)
  Selector1 : Selector  SampleTime=3.90625e-09  IndexOptions=Index vector (dialog)  Indices=double(7)  OutputSizes=double(1)
  Selector2 : Selector  SampleTime=3.90625e-09  IndexOptions=Index vector (dialog)  Indices=double(6)  OutputSizes=double(1)
  Selector3 : Selector  SampleTime=3.90625e-09  IndexOptions=Index vector (dialog)  Indices=double(5)  OutputSizes=double(1)
  Selector4 : Selector  SampleTime=3.90625e-09  IndexOptions=Index vector (dialog)  Indices=double(4)  OutputSizes=double(1)
  Selector5 : Selector  SampleTime=3.90625e-09  IndexOptions=Index vector (dialog)  Indices=double(3)  OutputSizes=double(1)
  Selector6 : Selector  SampleTime=3.90625e-09  IndexOptions=Index vector (dialog)  Indices=double(2)  OutputSizes=double(1)
  Selector7 : Selector  SampleTime=3.90625e-09  IndexOptions=Index vector (dialog)  Indices=double(1)  OutputSizes=double(1)
  SSR : Outport
  wires:
  Bit Concat/1 -> SSR/1
  Selector0/1 -> Bit Concat/1
  Selector1/1 -> Bit Concat/2
  Selector2/1 -> Bit Concat/3
  Selector3/1 -> Bit Concat/4
  Selector4/1 -> Bit Concat/5
  Selector5/1 -> Bit Concat/6
  Selector6/1 -> Bit Concat/7
  Selector7/1 -> Bit Concat/8
  Vector/1 -> Selector7/1, Selector6/1, Selector5/1, Selector4/1, Selector3/1, Selector2/1, Selector1/1, Selector0/1

== system gm_spectrum_analyser/Spectrum Analyser/Spectrum Analyser/Spectrum Analyser Core/SSR Subset Converter/SSR Serializer Real/SSR to Vector ==
  SSR : Inport  OutDataTypeStr=fixdt(0, 128, 0)  PortDimensions=1  SampleTime=3.90625e-09
  Bit Slice0 : hdlsllib/Logic and Bit Operations/Bit Slice  lidx=double(15)  ridx=double(0)
      settings: SourceProductBaseCode=SL
  Bit Slice1 : hdlsllib/Logic and Bit Operations/Bit Slice  lidx=double(31)  ridx=double(16)
      settings: SourceProductBaseCode=SL
  Bit Slice2 : hdlsllib/Logic and Bit Operations/Bit Slice  lidx=double(47)  ridx=double(32)
      settings: SourceProductBaseCode=SL
  Bit Slice3 : hdlsllib/Logic and Bit Operations/Bit Slice  lidx=double(63)  ridx=double(48)
      settings: SourceProductBaseCode=SL
  Bit Slice4 : hdlsllib/Logic and Bit Operations/Bit Slice  lidx=double(79)  ridx=double(64)
      settings: SourceProductBaseCode=SL
  Bit Slice5 : hdlsllib/Logic and Bit Operations/Bit Slice  lidx=double(95)  ridx=double(80)
      settings: SourceProductBaseCode=SL
  Bit Slice6 : hdlsllib/Logic and Bit Operations/Bit Slice  lidx=double(111)  ridx=double(96)
      settings: SourceProductBaseCode=SL
  Bit Slice7 : hdlsllib/Logic and Bit Operations/Bit Slice  lidx=double(127)  ridx=double(112)
      settings: SourceProductBaseCode=SL
  concatenate : Concatenate  NumInputs=8
  Vector : Outport
  wires:
  Bit Slice0/1 -> concatenate/1
  Bit Slice1/1 -> concatenate/2
  Bit Slice2/1 -> concatenate/3
  Bit Slice3/1 -> concatenate/4
  Bit Slice4/1 -> concatenate/5
  Bit Slice5/1 -> concatenate/6
  Bit Slice6/1 -> concatenate/7
  Bit Slice7/1 -> concatenate/8
  concatenate/1 -> Vector/1
  SSR/1 -> Bit Slice7/1, Bit Slice6/1, Bit Slice5/1, Bit Slice4/1, Bit Slice3/1, Bit Slice2/1, Bit Slice1/1, Bit Slice0/1

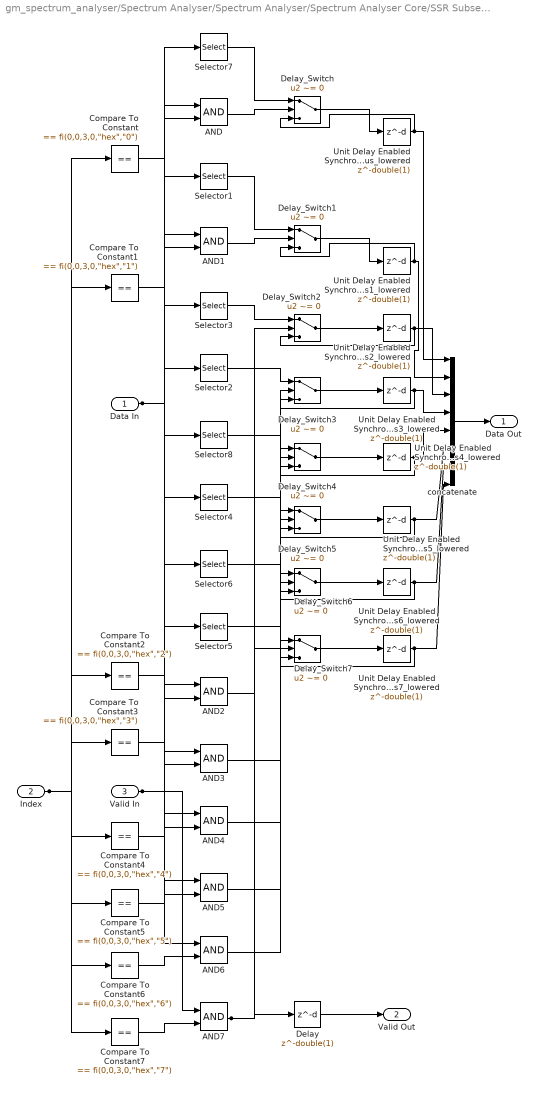
== system gm_spectrum_analyser/Spectrum Analyser/Spectrum Analyser/Spectrum Analyser Core/SSR Subset Converter/SSR Serializer Real/SSR1 to SSR8 ==
  Data In : Inport  OutDataTypeStr=uint16  PortDimensions=[8]  SampleTime=3.90625e-09
  Index : Inport  Port=2  OutDataTypeStr=fixdt(0, 3, 0)  PortDimensions=1  SampleTime=3.90625e-09
  Valid In : Inport  Port=3  OutDataTypeStr=boolean  PortDimensions=1  SampleTime=3.90625e-09
  AND{,1..7} (8 alike) : Logic  AllPortsSameDT=off  OutDataTypeStr=boolean  SampleTime=3.90625e-09
  Compare To Constant : simulink/Logic and Bit Operations/Compare To Constant  relop===  const="fi(0,0,3,0,\"hex\",\"0\")"  OutDataTypeStr=boolean
  Compare To Constant1 : simulink/Logic and Bit Operations/Compare To Constant  relop===  const="fi(0,0,3,0,\"hex\",\"1\")"  OutDataTypeStr=boolean
  Compare To Constant2 : simulink/Logic and Bit Operations/Compare To Constant  relop===  const="fi(0,0,3,0,\"hex\",\"2\")"  OutDataTypeStr=boolean
  Compare To Constant3 : simulink/Logic and Bit Operations/Compare To Constant  relop===  const="fi(0,0,3,0,\"hex\",\"3\")"  OutDataTypeStr=boolean
  Compare To Constant4 : simulink/Logic and Bit Operations/Compare To Constant  relop===  const="fi(0,0,3,0,\"hex\",\"4\")"  OutDataTypeStr=boolean
  Compare To Constant5 : simulink/Logic and Bit Operations/Compare To Constant  relop===  const="fi(0,0,3,0,\"hex\",\"5\")"  OutDataTypeStr=boolean
  Compare To Constant6 : simulink/Logic and Bit Operations/Compare To Constant  relop===  const="fi(0,0,3,0,\"hex\",\"6\")"  OutDataTypeStr=boolean
  Compare To Constant7 : simulink/Logic and Bit Operations/Compare To Constant  relop===  const="fi(0,0,3,0,\"hex\",\"7\")"  OutDataTypeStr=boolean
  Delay : Delay  DelayLength=double(1)  InitialCondition=0  SampleTime=3.90625e-09
  Delay_Switch{,1..7} (8 alike) : Switch  Criteria=u2 ~= 0  Threshold=double(0)  OutDataTypeStr=uint16  SampleTime=3.90625e-09
  Selector{1..8} (8 alike) : Selector  IndexMode=Zero-based  SampleTime=3.90625e-09  IndexOptions=Index vector (dialog)  Indices=double(0)  OutputSizes=double(1)
  Unit Delay Enabled Synchronous1_lowered : Delay  DelayLength=double(1)  InitialCondition=0  SampleTime=3.90625e-09
  Unit Delay Enabled Synchronous2_lowered : Delay  DelayLength=double(1)  InitialCondition=0  SampleTime=3.90625e-09
  Unit Delay Enabled Synchronous3_lowered : Delay  DelayLength=double(1)  InitialCondition=0  SampleTime=3.90625e-09
  Unit Delay Enabled Synchronous4_lowered : Delay  DelayLength=double(1)  InitialCondition=0  SampleTime=3.90625e-09
  Unit Delay Enabled Synchronous5_lowered : Delay  DelayLength=double(1)  InitialCondition=0  SampleTime=3.90625e-09
  Unit Delay Enabled Synchronous6_lowered : Delay  DelayLength=double(1)  InitialCondition=0  SampleTime=3.90625e-09
  Unit Delay Enabled Synchronous7_lowered : Delay  DelayLength=double(1)  InitialCondition=0  SampleTime=3.90625e-09
  Unit Delay Enabled Synchronous_lowered : Delay  DelayLength=double(1)  InitialCondition=0  SampleTime=3.90625e-09
  concatenate : Concatenate  NumInputs=8
  Data Out : Outport
  Valid Out : Outport  Port=2
  wires:
  AND/1 -> Delay_Switch/2
  AND1/1 -> Delay_Switch1/2
  AND2/1 -> Delay_Switch2/2
  AND3/1 -> Delay_Switch3/2
  AND4/1 -> Delay_Switch4/2
  AND5/1 -> Delay_Switch5/2
  AND6/1 -> Delay_Switch6/2
  AND7/1 -> Delay/1, Delay_Switch7/2
  Compare To Constant/1 -> AND/2
  Compare To Constant1/1 -> AND1/2
  Compare To Constant2/1 -> AND2/2
  Compare To Constant3/1 -> AND3/2
  Compare To Constant4/1 -> AND4/2
  Compare To Constant5/1 -> AND5/2
  Compare To Constant6/1 -> AND6/2
  Compare To Constant7/1 -> AND7/2
  Delay/1 -> Valid Out/1
  Selector1/1 -> Delay_Switch1/1
  Selector2/1 -> Delay_Switch3/1
  Selector3/1 -> Delay_Switch2/1
  Selector4/1 -> Delay_Switch5/1
  Selector5/1 -> Delay_Switch7/1
  Selector6/1 -> Delay_Switch6/1
  Selector7/1 -> Delay_Switch/1
  Selector8/1 -> Delay_Switch4/1
  Unit Delay Enabled Synchronous_lowered/1 -> concatenate/1, Delay_Switch/3
  Unit Delay Enabled Synchronous1_lowered/1 -> concatenate/2, Delay_Switch1/3
  Unit Delay Enabled Synchronous2_lowered/1 -> concatenate/3, Delay_Switch2/3
  Unit Delay Enabled Synchronous3_lowered/1 -> concatenate/4, Delay_Switch3/3
  Unit Delay Enabled Synchronous4_lowered/1 -> concatenate/5, Delay_Switch4/3
  Unit Delay Enabled Synchronous5_lowered/1 -> concatenate/6, Delay_Switch5/3
  Unit Delay Enabled Synchronous6_lowered/1 -> concatenate/7, Delay_Switch6/3
  Unit Delay Enabled Synchronous7_lowered/1 -> concatenate/8, Delay_Switch7/3
  concatenate/1 -> Data Out/1
  Data In/1 -> Selector8/1, Selector7/1, Selector6/1, Selector5/1, Selector4/1, Selector3/1, Selector2/1, Selector1/1
  Index/1 -> Compare To Constant7/1, Compare To Constant6/1, Compare To Constant5/1, Compare To Constant4/1, Compare To Constant3/1, Compare To Constant2/1, Compare To Constant1/1, Compare To Constant/1
  Valid In/1 -> AND7/1, AND6/1, AND5/1, AND4/1, AND3/1, AND2/1, AND1/1, AND/1
  Delay_Switch/1 -> Unit Delay Enabled Synchronous_lowered/1
  Delay_Switch1/1 -> Unit Delay Enabled Synchronous1_lowered/1
  Delay_Switch2/1 -> Unit Delay Enabled Synchronous2_lowered/1
  Delay_Switch3/1 -> Unit Delay Enabled Synchronous3_lowered/1
  Delay_Switch4/1 -> Unit Delay Enabled Synchronous4_lowered/1
  Delay_Switch5/1 -> Unit Delay Enabled Synchronous5_lowered/1
  Delay_Switch6/1 -> Unit Delay Enabled Synchronous6_lowered/1
  Delay_Switch7/1 -> Unit Delay Enabled Synchronous7_lowered/1

== system gm_spectrum_analyser/Spectrum Analyser/Spectrum Analyser/Spectrum Analyser Core/SSR Subset Converter/SSR Serializer Real/SSR2 to SSR8 ==
  Data In : Inport  OutDataTypeStr=uint16  PortDimensions=[8]  SampleTime=3.90625e-09
  Index : Inport  Port=2  OutDataTypeStr=fixdt(0, 2, 0)  PortDimensions=1  SampleTime=3.90625e-09
  Valid In : Inport  Port=3  OutDataTypeStr=boolean  PortDimensions=1  SampleTime=3.90625e-09
  AND{,1..3} (4 alike) : Logic  AllPortsSameDT=off  OutDataTypeStr=boolean  SampleTime=3.90625e-09
  Compare To Constant10 : simulink/Logic and Bit Operations/Compare To Constant  relop===  const="fi(0,0,2,0,\"hex\",\"2\")"  OutDataTypeStr=boolean
  Compare To Constant11 : simulink/Logic and Bit Operations/Compare To Constant  relop===  const="fi(0,0,2,0,\"hex\",\"3\")"  OutDataTypeStr=boolean
  Compare To Constant8 : simulink/Logic and Bit Operations/Compare To Constant  relop===  const="fi(0,0,2,0,\"hex\",\"0\")"  OutDataTypeStr=boolean
  Compare To Constant9 : simulink/Logic and Bit Operations/Compare To Constant  relop===  const="fi(0,0,2,0,\"hex\",\"1\")"  OutDataTypeStr=boolean
  Delay : Delay  DelayLength=double(1)  InitialCondition=0  SampleTime=3.90625e-09
  Delay_Switch{,1..3} (4 alike) : Switch  Criteria=u2 ~= 0  Threshold=double(0)  OutDataTypeStr=uint16  SampleTime=3.90625e-09
  Selector{9..12} (4 alike) : Selector  IndexMode=Zero-based  SampleTime=3.90625e-09  IndexOptions=Index vector (dialog)  Indices=double([0 1])  OutputSizes=double(1)
  Unit Delay Enabled Synchronous1_lowered : Delay  DelayLength=double(1)  InitialCondition=0  SampleTime=3.90625e-09
  Unit Delay Enabled Synchronous2_lowered : Delay  DelayLength=double(1)  InitialCondition=0  SampleTime=3.90625e-09
  Unit Delay Enabled Synchronous3_lowered : Delay  DelayLength=double(1)  InitialCondition=0  SampleTime=3.90625e-09
  Unit Delay Enabled Synchronous_lowered : Delay  DelayLength=double(1)  InitialCondition=0  SampleTime=3.90625e-09
  concatenate : Concatenate  NumInputs=8
  t{,1..3} (4 alike) : Demux  Outputs=2
  Data Out : Outport
  Valid Out : Outport  Port=2
  wires:
  AND/1 -> Delay_Switch/2
  AND1/1 -> Delay_Switch1/2
  AND2/1 -> Delay_Switch2/2
  AND3/1 -> Delay/1, Delay_Switch3/2
  Compare To Constant10/1 -> AND2/2
  Compare To Constant11/1 -> AND3/2
  Compare To Constant8/1 -> AND/2
  Compare To Constant9/1 -> AND1/2
  Delay/1 -> Valid Out/1
  Selector10/1 -> Delay_Switch2/1
  Selector11/1 -> Delay_Switch3/1
  Selector12/1 -> Delay_Switch/1
  Selector9/1 -> Delay_Switch1/1
  Unit Delay Enabled Synchronous_lowered/1 -> t/1, Delay_Switch/3
  Unit Delay Enabled Synchronous1_lowered/1 -> t1/1, Delay_Switch1/3
  Unit Delay Enabled Synchronous2_lowered/1 -> t2/1, Delay_Switch2/3
  Unit Delay Enabled Synchronous3_lowered/1 -> t3/1, Delay_Switch3/3
  concatenate/1 -> Data Out/1
  t/1 -> concatenate/1
  t/2 -> concatenate/2
  t1/1 -> concatenate/3
  t1/2 -> concatenate/4
  t2/1 -> concatenate/5
  t2/2 -> concatenate/6
  t3/1 -> concatenate/7
  t3/2 -> concatenate/8
  Data In/1 -> Selector9/1, Selector12/1, Selector11/1, Selector10/1
  Index/1 -> Compare To Constant9/1, Compare To Constant8/1, Compare To Constant11/1, Compare To Constant10/1
  Valid In/1 -> AND3/1, AND2/1, AND1/1, AND/1
  Delay_Switch/1 -> Unit Delay Enabled Synchronous_lowered/1
  Delay_Switch1/1 -> Unit Delay Enabled Synchronous1_lowered/1
  Delay_Switch2/1 -> Unit Delay Enabled Synchronous2_lowered/1
  Delay_Switch3/1 -> Unit Delay Enabled Synchronous3_lowered/1
